simulink model "fuzzy"  (R2019a)
settings: Solver=VariableStepAuto  StartTime=0.0  StopTime=20  RelTol=1e-3
undefined symbols (not defined in the file): J, Ke_Phi, Km_Phi, La, Ra
libraries: fuzblock x1
settings Model: Creator=Chi Tuyen  LastModifiedBy=Chi Tuyen

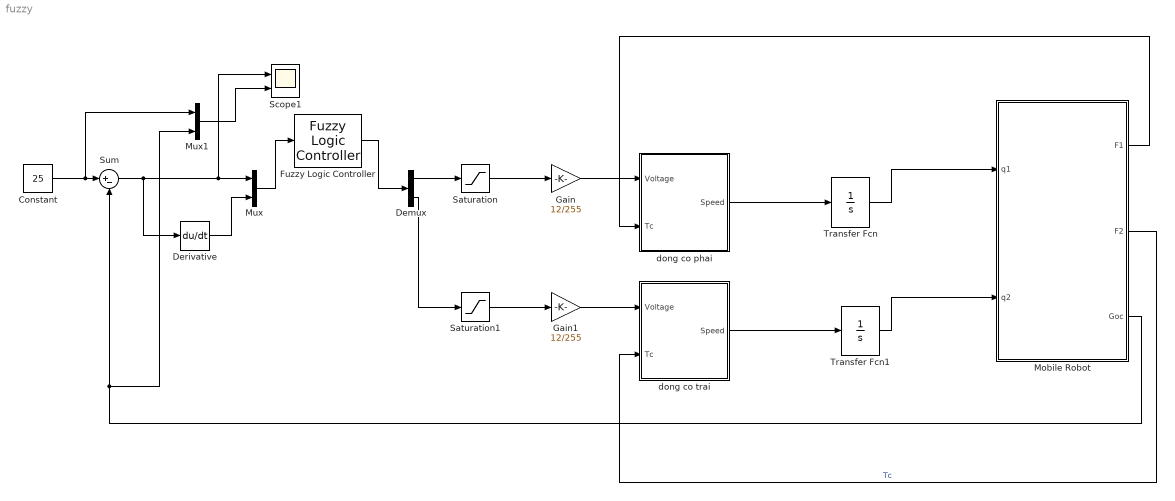
== system fuzzy ==
  Constant : Constant  Value=25
  Demux : Demux  Outputs=2
  Derivative : Derivative
  Fuzzy Logic Controller : fuzblock/Fuzzy Logic  Controller  FIS=fuzzy_dc4  OutputSampleNumber=101  DataType=double  FuzzifiedInputs=off  RuleFiringStrengths=off  RuleOutputs=off  AggregatedOutputs=off  SimulateUsing=Interpreted execution  OutOfRangeInputValueMessage=warning  NoRuleFiredMessage=warning  EmptyOutputFuzzySetMessage=warning
  Gain : Gain  Gain=12/255
  Gain1 : Gain  Gain=12/255
  Mobile Robot : Subsystem
  Mux : Mux  Inputs=2
  Mux1 : Mux  Inputs=2
  Saturation : Saturate
  Saturation1 : Saturate
  Scope1 : Scope  NumInputPorts=2
  Sum : Sum  Inputs=|+-
  Transfer Fcn : TransferFcn  Denominator=[1 0]
  Transfer Fcn1 : TransferFcn  Denominator=[1 0]
  "dong co phai " : Subsystem
  "dong co trai " : Subsystem
  wires:
  Constant/1 -> Mux1/1, Sum/1
  Sum/1 -> Mux/1, Scope1/1, Derivative/1
  Demux/2 -> Saturation1/1
  Transfer Fcn/1 -> Mobile Robot/1(q1)
  Transfer Fcn1/1 -> Mobile Robot/2(q2)
  "dong co trai "/1("Speed ") -> Transfer Fcn1/1
  "dong co phai "/1("Speed ") -> Transfer Fcn/1
  Demux/1 -> Saturation/1
  Derivative/1 -> Mux/2
  Fuzzy Logic Controller/1 -> Demux/1
  Mux/1 -> Fuzzy Logic Controller/1
  Mobile Robot/3("Goc ") -> Sum/2, Mux1/2
  Mobile Robot/1(F1) -> "dong co phai "/2("Tc ")
  Mobile Robot/2(F2) -> "dong co trai "/2("Tc ")  "Tc"
  Mux1/1 -> Scope1/2
  Saturation/1 -> Gain/1
  Saturation1/1 -> Gain1/1
  Gain/1 -> "dong co phai "/1("Voltage ")
  Gain1/1 -> "dong co trai "/1("Voltage ")

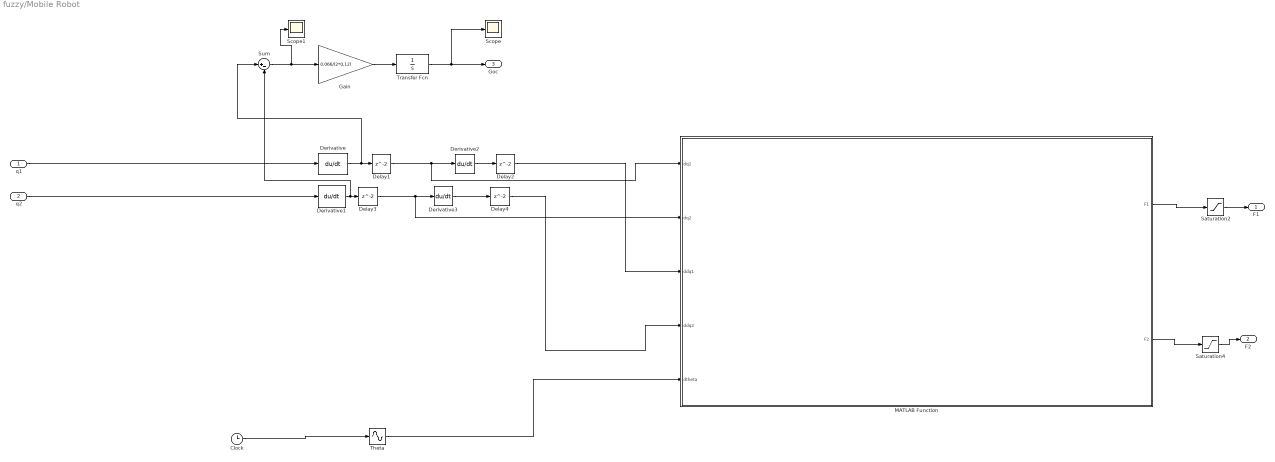
== system fuzzy/Mobile Robot ==
  q1 : Inport
  q2 : Inport  Port=2
  Clock : Clock
      settings: Decimation=5
  Delay{1..4} (4 alike) : Delay  SampleTime=0.001
  Derivative{,1..3} (4 alike) : Derivative
  Gain : Gain  Gain=0.066/(2*0.12)
  MATLAB Function : MATLAB Function  TreatAsAtomicUnit=on
  Saturation2 : Saturate
  Saturation4 : Saturate
  Scope : Scope
  Scope1 : Scope
  Sum : Sum  Inputs=|+-
  Theta : Sin  TimeSource=Use external signal  Frequency=60  Phase=30  SampleTime=0
  Transfer Fcn : TransferFcn  Denominator=[1 0]
  F1 : Outport
  F2 : Outport  Port=2
  "Goc " : Outport  Port=3
  wires:
  q2/1 -> Derivative1/1
  Derivative1/1 -> Sum/2, Delay3/1
  Derivative/1 -> Sum/1, Delay1/1
  Derivative3/1 -> Delay4/1
  q1/1 -> Derivative/1
  Delay1/1 -> MATLAB Function/1(dq1), Derivative2/1
  Derivative2/1 -> Delay2/1
  Delay3/1 -> MATLAB Function/2(dq2), Derivative3/1
  Clock/1 -> Theta/1
  Theta/1 -> MATLAB Function/5(dtheta)
  Delay2/1 -> MATLAB Function/3(ddq1)
  Delay4/1 -> MATLAB Function/4(ddq2)
  Saturation2/1 -> F1/1
  MATLAB Function/1(F1) -> Saturation2/1
  MATLAB Function/2(F2) -> Saturation4/1
  Saturation4/1 -> F2/1
  Gain/1 -> Transfer Fcn/1
  Sum/1 -> Scope1/1, Gain/1
  Transfer Fcn/1 -> "Goc "/1, Scope/1

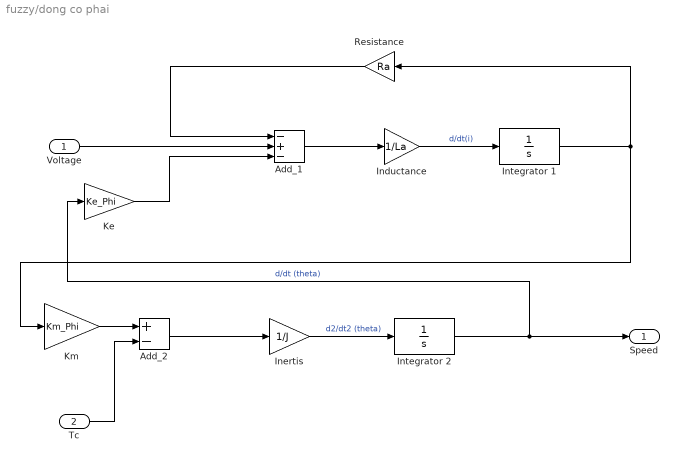
== system fuzzy/dong co phai  ==
  "Voltage " : Inport
  "Tc " : Inport  Port=2
  "Add_1 " : Sum  Inputs=-+-
  "Add_2 " : Sum  Inputs=+-
  "Inductance " : Gain  Gain=1/La
  "Inertis " : Gain  Gain=1/J
  "Integrator 1 " : TransferFcn  Denominator=[1 0]
  "Integrator 2 " : TransferFcn  Denominator=[1 0]
  "Ke " : Gain  Gain=Ke_Phi
  "Km " : Gain  Gain=Km_Phi
  Resistance : Gain  Gain=Ra
  "Speed " : Outport
  wires:
  "Ke "/1 -> "Add_1 "/3
  Resistance/1 -> "Add_1 "/1
  "Voltage "/1 -> "Add_1 "/2
  "Add_1 "/1 -> "Inductance "/1
  "Add_2 "/1 -> "Inertis "/1
  "Km "/1 -> "Add_2 "/1
  "Integrator 2 "/1 -> "Ke "/1, "Speed "/1  "d/dt (theta)"
  "Inertis "/1 -> "Integrator 2 "/1  "d2/dt2 (theta)"
  "Integrator 1 "/1 -> "Km "/1, Resistance/1
  "Inductance "/1 -> "Integrator 1 "/1  "d/dt(i)"
  "Tc "/1 -> "Add_2 "/2

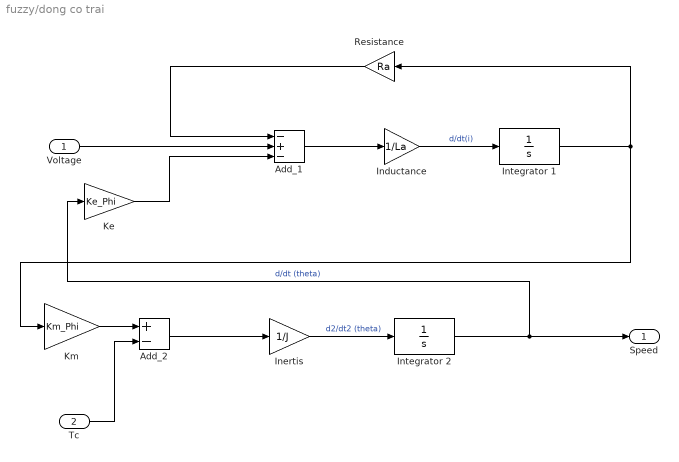
== system fuzzy/dong co trai  ==
  "Voltage " : Inport
  "Tc " : Inport  Port=2
  "Add_1 " : Sum  Inputs=-+-
  "Add_2 " : Sum  Inputs=+-
  "Inductance " : Gain  Gain=1/La
  "Inertis " : Gain  Gain=1/J
  "Integrator 1 " : TransferFcn  Denominator=[1 0]
  "Integrator 2 " : TransferFcn  Denominator=[1 0]
  "Ke " : Gain  Gain=Ke_Phi
  "Km " : Gain  Gain=Km_Phi
  Resistance : Gain  Gain=Ra
  "Speed " : Outport
  wires:
  "Ke "/1 -> "Add_1 "/3
  Resistance/1 -> "Add_1 "/1
  "Voltage "/1 -> "Add_1 "/2
  "Add_1 "/1 -> "Inductance "/1
  "Add_2 "/1 -> "Inertis "/1
  "Km "/1 -> "Add_2 "/1
  "Integrator 2 "/1 -> "Ke "/1, "Speed "/1  "d/dt (theta)"
  "Inertis "/1 -> "Integrator 2 "/1  "d2/dt2 (theta)"
  "Integrator 1 "/1 -> "Km "/1, Resistance/1
  "Inductance "/1 -> "Integrator 1 "/1  "d/dt(i)"
  "Tc "/1 -> "Add_2 "/2

== matlab function fuzzy/Mobile Robot/MATLAB Function ==
  data: dq1 input; dq2 input; ddq1 input; ddq2 input; dtheta input; F1 output; F2 output
function [F1,F2]= fcn(dq1,dq2,ddq1,ddq2,dtheta)
IW=1;
R=0.5;
mc=5;
mw=0.2;
L=10;
d=5;
Ic=2;
Im=1;

dq=[dq1;dq2];
ddq=[ddq1;ddq2];
m=mc+2*mw;
I=Ic+mc*d^2+2*mw*L^2+2*Im;

M=[IW+(R^2)*(m*L^2+I)/(4*L),(R^2)*(m*L^2-I)/(4*L);
    (R^2)*(m*L^2-I)/(4*L) ,IW+(R^2)*(m*L^2+I)/(4*L)];
    
V=[0, (R^2)*(mc*dtheta)/(2*L);
  -(R^2)*(mc*dtheta)/(2*L),0];

F=M*ddq+V*dq;
F1=F(1,1);
F2=F(2,1);
